simulink subsystem "altitude_control"  (R2021a)
settings: Solver=VariableStepAuto  StartTime=0.0  StopTime=10.0  RelTol=1e-3
undefined symbols (not defined in the file or in its folder): Ts_alt
settings Model: Creator=EpEp  LastModifiedBy=EpEp

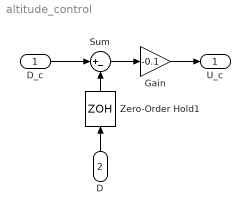
== system altitude_control ==
  D_c : Inport
  D : Inport  Port=2
  Gain : Gain  Gain=-0.1
  Sum : Sum  Inputs=|+-
  Zero-Order Hold1 : ZeroOrderHold  SampleTime=Ts_alt
  U_c : Outport
  wires:
  Gain/1 -> U_c/1
  D_c/1 -> Sum/1
  Sum/1 -> Gain/1
  Zero-Order Hold1/1 -> Sum/2
  D/1 -> Zero-Order Hold1/1
